simulink model "RTCDEMO"  (R2014b)
settings: Solver=FixedStepDiscrete  StartTime=0.0  StopTime=10.0  FixedStep=0.5  RelTol=1e-3
PreLoadFcn:
  | Hyo_customization
undefined symbols (not defined in the file): _IntStatus_CFD, _MalTrig, _Reset, _Start, _Status_CLK_STS, _Status_RUNC, _Stop, _Update, _Update_Calibration, autocal, CFD, CLK_STS, noparam, regbit, Reset, RTC, RUNC, s6j3200_RTC, start, Start, Stop, Update
libraries: periblklib x11
settings Model: Creator=Hyowinner  LastModifiedBy=sunzx.fnst
settings OptimizationCC: InlineParams=on  OptimizeModelRefInitCode=on  LifeSpan=1
settings HardwareCC: ProdLargestAtomicInteger=Integer  ProdLargestAtomicFloat=Float  ProdIntDivRoundTo=Zero  ProdEndianess=LittleEndian  ProdHWDeviceType=CYPRESS->ARM Cortex-R5
settings RTWCC: SystemTargetFile=Hyo.tlc  GenCodeOnly=on  MakeCommand=none  GenerateMakefile=off  TemplateMakefile=none  Description=System Target File for S6J3200 Series MCU Target  GenerateReport=on  ProcessScript=Hyo_make_rtw_hook  IncludeHyperlinkInReport=on  LaunchReport=on
settings CodeAppCC: IgnoreCustomStorageClasses=off
settings STFCustomTargetCC: ModelReferenceCompliant=off  IncludeMdlTerminateFcn=off  CombineOutputUpdateFcns=on  ERTFirstTimeCompliant=on  ERTCustomFileBanners=on  SupportContinuousTime=off  SupportNonInlinedSFcns=off  MATLABClassNameForMDSCustomization=Simulink.SoftwareTarget.ERTCustomization  GRTInterface=off  SystemTargetFile=Hyo.tlc
settings ERTTargetCC: ModelReferenceCompliant=off  ParMdlRefBuildCompliant=off  CompOptLevelCompliant=off  ConcurrentExecutionCompliant=off  IncludeMdlTerminateFcn=off  ModelStepFunctionPrototypeControlCompliant=off  CPPClassGenCompliant=off  InlinedParameterPlacement=NonHierarchical  ERTSrcFileBannerTemplate=Hyo_code_template.cgt  ERTHdrFileBannerTemplate=Hyo_code_template.cgt  ERTDataSrcFileTemplate=Hyo_code_template.cgt  ERTDataHdrFileTemplate=Hyo_code_template.cgt  ERTCustomFileTemplate=Hyo_file_process.tlc  EnableUserReplacementTypes=on

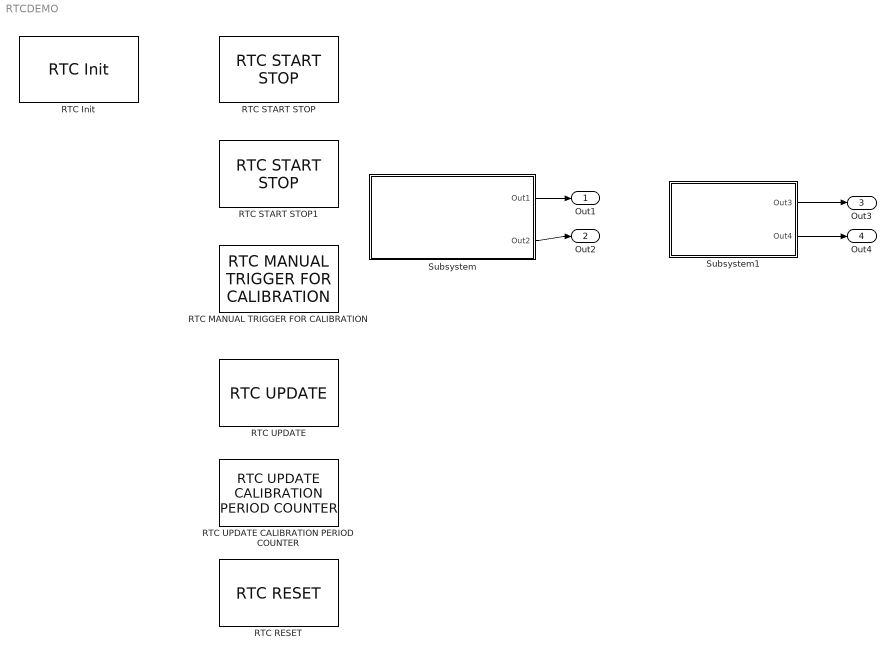
== system RTCDEMO ==
  RTC Init : periblklib/Real Time Clock/RTC Init  g_pv=s6j3200_RTC.h,RTC,_Init;daybit,0;hour,0;minute,0;second,0;subsec,0;scalecalval,Multiply by 2;clkselcali,Sub clock (CLK_SUB);encalvalupdt,off;autocal,off;calclkprd,267;caldur,0x07A120;caltrigcntval,0;debug,off;clksel4rtc,Main clock (CLK_MAIN/2);clcswmode,Immediate switch;caldoneinten,on;calfaildetinten,on;outputen,used as a General-purpose I/O or for another peripheral block;dayinten,on;hourinten,on;mininten,on;secinten,on;subsecinten,on;wot,P3_08;
  RTC MANUAL TRIGGER FOR CALIBRATION : periblklib/Real Time Clock/RTC MANUAL TRIGGER FOR CALIBRATION  g_pv=s6j3200_RTC.h,RTC,_MalTrig;autocal,off;
  RTC RESET : periblklib/Real Time Clock/RTC RESET  g_pv=s6j3200_RTC.h,RTC,_Reset;noparam,Reset;
  RTC START STOP : periblklib/Real Time Clock/RTC START STOP  g_pv=s6j3200_RTC.h,RTC,_Start;start,Start;
  RTC START STOP1 : periblklib/Real Time Clock/RTC START STOP  g_pv=s6j3200_RTC.h,RTC,_Stop;start,Stop;
  RTC UPDATE : periblklib/Real Time Clock/RTC UPDATE  g_pv=s6j3200_RTC.h,RTC,_Update;noparam,Update;
  RTC UPDATE CALIBRATION PERIOD COUNTER : periblklib/Real Time Clock/RTC UPDATE CALIBRATION PERIOD COUNTER  g_pv=s6j3200_RTC.h,RTC,_Update_Calibration;noparam,Update;
  Subsystem : Subsystem  TreatAsAtomicUnit=on  SystemSampleTime=1
  Subsystem1 : Subsystem  TreatAsAtomicUnit=on  SystemSampleTime=2
  Out1 : Outport
  Out2 : Outport  Port=2
  Out3 : Outport  Port=3
  Out4 : Outport  Port=4
  wires:
  Subsystem/1(Out1) -> Out1/1
  Subsystem/2(Out2) -> Out2/1
  Subsystem1/1(Out3) -> Out3/1
  Subsystem1/2(Out4) -> Out4/1

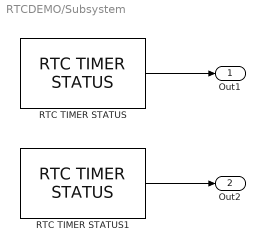
== system RTCDEMO/Subsystem ==
  RTC TIMER STATUS : periblklib/Real Time Clock/RTC TIMER STATUS  g_pv=s6j3200_RTC.h,RTC,_Status_CLK_STS;regbit,CLK_STS;
  RTC TIMER STATUS1 : periblklib/Real Time Clock/RTC TIMER STATUS  g_pv=s6j3200_RTC.h,RTC,_Status_RUNC;regbit,RUNC;
  Out1 : Outport
  Out2 : Outport  Port=2
  wires:
  RTC TIMER STATUS/1 -> Out1/1
  RTC TIMER STATUS1/1 -> Out2/1

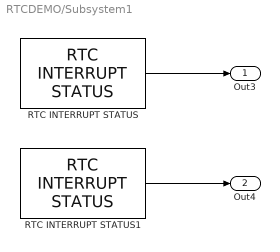
== system RTCDEMO/Subsystem1 ==
  RTC INTERRUPT STATUS : periblklib/Real Time Clock/RTC INTERRUPT STATUS  g_pv=s6j3200_RTC.h,RTC,_IntStatus_CFD;regbit,CFD;
  RTC INTERRUPT STATUS1 : periblklib/Real Time Clock/RTC INTERRUPT STATUS  g_pv=s6j3200_RTC.h,RTC,_IntStatus_CFD;regbit,CFD;
  Out3 : Outport
  Out4 : Outport  Port=2
  wires:
  RTC INTERRUPT STATUS/1 -> Out3/1
  RTC INTERRUPT STATUS1/1 -> Out4/1
